simulink model "PenulumAccelerationInput"  (R2017b)
settings: Solver=ode45  StartTime=0.0  StopTime=20  RelTol=1e-9
InitFcn:
  | Init_Simple_Pemdulum
undefined symbols (not defined in the file): g, Kda, Kp, L, omega0, zeta
libraries: simulink x1
settings Model: Creator=oe  LastModifiedBy=oe

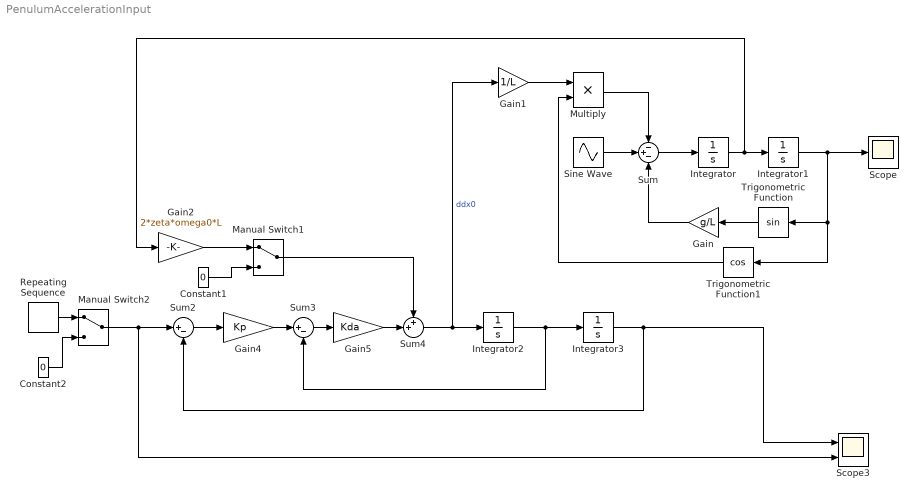
== system PenulumAccelerationInput ==
  Constant1 : Constant  Value=0
  Constant2 : Constant  Value=0
  Gain : Gain  Gain=g/L
  Gain1 : Gain  Gain=1/L
  Gain2 : Gain  Gain=2*zeta*omega0*L
  Gain4 : Gain  Gain=Kp
  Gain5 : Gain  Gain=Kda
  Integrator : Integrator
  Integrator1 : Integrator  InitialCondition=0.1
  Integrator2 : Integrator
  Integrator3 : Integrator
  Manual Switch1 : ManualSwitch
  Manual Switch2 : ManualSwitch
  Multiply : Product  Inputs=**
  Repeating Sequence : simulink/Sources/Repeating Sequence  rep_seq_t=[0 5 10 15 20]  rep_seq_y=[-0.5 0.5 -0.5 0.5 -0.5]
  Scope : Scope
  Scope3 : Scope  NumInputPorts=2
  Sine Wave : Sin  Amplitude=0  SampleTime=0
  Sum : Sum  Inputs=-+-
  Sum2 : Sum  Inputs=|+-
  Sum3 : Sum  Inputs=|+-
  Sum4 : Sum  Inputs=++|
  Trigonometric Function : Trigonometry
  Trigonometric Function1 : Trigonometry  Operator=cos
  wires:
  Integrator/1 -> Gain2/1, Integrator1/1
  Integrator1/1 -> Trigonometric Function1/1, Trigonometric Function/1, Scope/1
  Trigonometric Function/1 -> Gain/1
  Sum/1 -> Integrator/1
  Trigonometric Function1/1 -> Multiply/2
  Gain1/1 -> Multiply/1
  Multiply/1 -> Sum/1
  Gain/1 -> Sum/3
  Sine Wave/1 -> Sum/2
  Integrator2/1 -> Sum3/2, Integrator3/1
  Integrator3/1 -> Sum2/2, Scope3/1
  Sum2/1 -> Gain4/1
  Gain2/1 -> Manual Switch1/1
  Constant1/1 -> Manual Switch1/2
  Repeating Sequence/1 -> Manual Switch2/1
  Manual Switch2/1 -> Scope3/2, Sum2/1
  Constant2/1 -> Manual Switch2/2
  Gain4/1 -> Sum3/1
  Sum3/1 -> Gain5/1
  Manual Switch1/1 -> Sum4/1
  Gain5/1 -> Sum4/2
  Sum4/1 -> Gain1/1, Integrator2/1  "ddx0"
